simulink model "Master_compact"  (R2016b)
settings: Solver=FixedStepDiscrete  StartTime=0.0  StopTime=3000e-6  FixedStep=10e-9  RelTol=1e-3
undefined symbols (not defined in the file): plecs
libraries: hdlsllib x2, simulink x2, modelsimlib x1
settings Model: Creator=pzaehner  LastModifiedBy=pzaehner

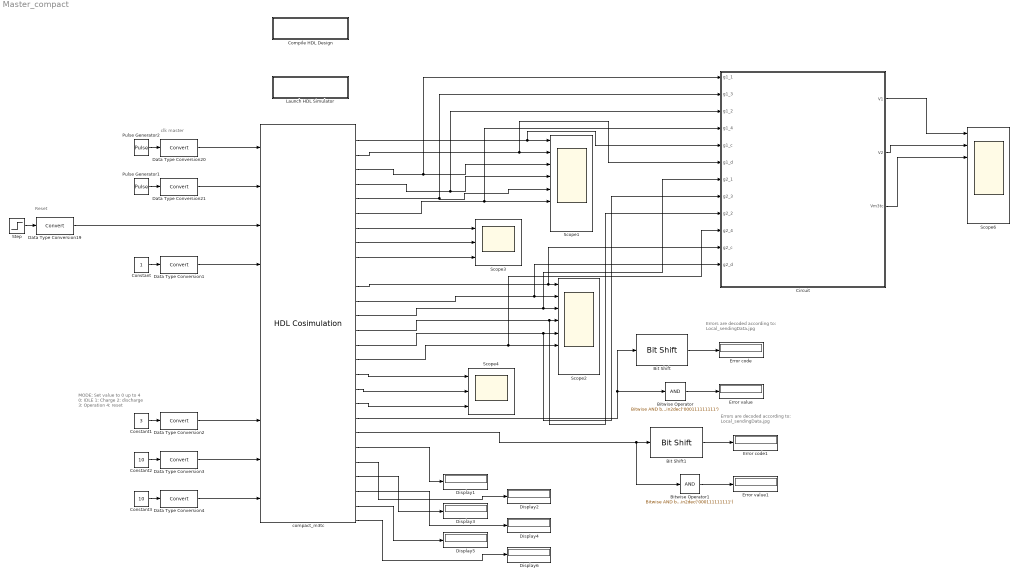
== system Master_compact ==
  note: clk master
  note: Reset
  note: MODE:
      | Set value to 0 up to 4
      | 0: IDLE
      | 1: Charge
      | 2: discharge
      | 3: Operation
      | 4: reset
  note: Errors are decoded according to:
      | Local_sendingData.jpg
  note: Errors are decoded according to:
      | Local_sendingData.jpg
  Bit Shift : hdlsllib/HDL Operations/Bit Shift  mode=Shift Right Logical  N=9
  Bit Shift1 : hdlsllib/HDL Operations/Bit Shift  mode=Shift Right Logical  N=9
  Bitwise Operator : simulink/Logic and Bit Operations/Bitwise Operator  logicop=AND  UseBitMask=on  BitMask=bin2dec('000111111111')  BitMaskRealWorld=Stored Integer
  Bitwise Operator1 : simulink/Logic and Bit Operations/Bitwise Operator  logicop=AND  UseBitMask=on  BitMask=bin2dec('000111111111')  BitMaskRealWorld=Stored Integer
  Circuit : Subsystem  LoadFcn=plecs('sl', 200);  InitFcn=plecs('sl', 214);  StartFcn=plecs('sl', 208);  StopFcn=plecs('sl', 209);  mask(PlecsCircuit){PLECSData=<binary blob, 7016 chars, not shown>}
      mask prompts: PLECSData "PLECS Data (Do not delete or modify!)"
      mask init:
      | % PLACE CUSTOM INITIALIZATIONS ABOVE
      | % DO NOT REMOVE
      | plecs('sl', 215);
      | % DO NOT REMOVE
      settings: CopyFcn=plecs('sl', 203);  DeleteFcn=plecs('sl', 205);  UndoDeleteFcn=plecs('sl', 206);  PreSaveFcn=plecs('sl', 211);  PostSaveFcn=plecs('sl', 201);  NameChangeFcn=plecs('sl', 210);  DestroyFcn=plecs('sl', 207);  PreCopyFcn=plecs('sl', 216);  OpenFcn=plecs('sl', 202);  ErrorFcn=plerrorfcn
      mask Help: web(['file:///' fullfile(plecsdoc, 'creatingacircuit.html')])
      mask Display: disp('PLECS\nCircuit')
  Compile HDL Design : Subsystem
      settings: OpenFcn=eval('compile_hdl_design_compact_m3tc');
      mask Display: disp(['Double-Click to' char(10) 'compile HDL files'])
  Constant : Constant  SampleTime=10e-9
  Constant1 : Constant  Value=3  SampleTime=10e-9
  Constant2 : Constant  Value=10  SampleTime=10e-9
  Constant3 : Constant  Value=10  SampleTime=10e-9
  Data Type Conversion{1..4,19..21} (7 alike) : DataTypeConversion
  Display{1..6} (6 alike) : Display
  Error code : Display
  Error code1 : Display
  Error value : Display
  Error value1 : Display
  Launch HDL Simulator : Subsystem
      settings: OpenFcn=eval('launch_hdl_simulator_compact_m3tc');
      mask Display: disp(['Double-Click to' char(10) 'launch HDL simulator'])
  Pulse Generator1 : DiscretePulseGenerator  PulseType=Time based  Period=20e-9  PulseWidth=50  PhaseDelay=10e-9
  Pulse Generator2 : DiscretePulseGenerator  PulseType=Time based  Period=20e-9  PulseWidth=50  PhaseDelay=10e-9
  Scope1 : Scope  NumInputPorts=8
  Scope2 : Scope  NumInputPorts=8
  Scope3 : Scope  NumInputPorts=3
  Scope4 : Scope  NumInputPorts=3
  Scope6 : Scope  NumInputPorts=8
  Step : Step  Time=100e-9  SampleTime=10e-9
  compact_m3tc : modelsimlib/HDL Cosimulation  PortPaths=/compact_m3tc/CLK_Master;/compact_m3tc/optical_Clk_1;/compact_m3tc/nreset;/compact_m3tc/HIGH_Input;/compact_m3tc/masterCurrentMeas;/compact_m3tc/masterCurrentRef;/compact_m3tc/masterVOLT;/compact_m3tc/MODE_put_to_3;/compact_m3tc/Number_12_bit3;/compact_m3tc/Number_8_bit;/compact_m3tc/optical_fault_1;/compact_m3tc/gate_c_1;/compact_m3tc/gate_d_1;/compact_m3tc/gate_1_1;/compact_m3tc/gate_2_1;/compact_m3tc/gate_3_1;/compact_m3tc/gate_4_1;/compact_m3tc/rst_c_1;/compact_m3tc/rst_d_1;/compact_m3tc/rst_overall_1;/compact_m3tc/optical_fault_2;/compact_m3tc/gate_c_2;/compact_m3tc/gate_d_2;/compact_m3tc/gate_1_2;/compact_m3tc/gate_2_2;/compact_m3tc/gate_3_2;/compact_m3tc/gate_4_2;/compact_m3tc/rst_c_2;/compact_m3tc/rst_d_2;/compact_m3tc/rst_overall_2;/compact_m3tc/outFAULT_1;/compact_m3tc/outFAULT_2;/compact_m3tc/outTempHS_1;/compact_m3tc/outTempHS_2;/compact_m3tc/outTempIGBT_1;/compact_m3tc/outTempIGBT_2;/compact_m3tc/outVOLT_1;/compact_m3tc/outVOLT_2;  PortModes=[1 1 1 1 1 1 1 1 1 1 2 2 2 2 2 2 2 2 2 2 2 2 2 2 2 2 2 2 2 2 2 2 2 2 2 2 2 2 ]  PortTimes=[-1,-1,-1,-1,-1,-1,-1,-1,-1,-1,10e-9,10e-9,10e-9,10e-9,10e-9,10e-9,10e-9,10e-9,10e-9,10e-9,10e-9,10e-9,10e-9,10e-9,10e-9,10e-9,10e-9,10e-9,10e-9,10e-9,10e-9,10e-9,10e-9,10e-9,10e-9,10e-9,10e-9,10e-9]  PortSigns=[-1,-1,-1,-1,-1,-1,-1,-1,-1,-1,-1,-1,-1,-1,-1,-1,-1,-1,-1,-1,-1,-1,-1,-1,-1,-1,-1,-1,-1,-1,-1,-1,-1,-1,-1,-1,-1,-1,]  PortFracLengths=[0,0,0,0,0,0,0,0,0,0,0,0,0,0,0,0,0,0,0,0,0,0,0,0,0,0,0,0,0,0,0,0,0,0,0,0,0,0]  CommLocal=on  CommSharedMemory=off  CommPortNumber=49294  CommShowInfo=on  ClockModes=[]  ClockTimes=[]  TclPostSimCommand="puts \"done\";"  TimingMode=s  TimingScaleFactor=1  idxCellArray={'UNUSED_VAR'}  CosimBypass=Full Simulation  AllowDirectFeedthrough=on  ProductName=EDA Simulator Link MQ  RunAutoTimescale=on  PreRunTime=0  PreRunTimeUnit=ns
  wires:
  Data Type Conversion19/1 -> compact_m3tc/3
  Step/1 -> Data Type Conversion19/1
  Pulse Generator2/1 -> Data Type Conversion20/1
  Pulse Generator1/1 -> Data Type Conversion21/1
  Data Type Conversion21/1 -> compact_m3tc/2
  Circuit/1(V1) -> Scope6/1
  Circuit/2(V2) -> Scope6/2
  Bit Shift/1 -> Error code/1
  Bitwise Operator/1 -> Error value/1
  Bit Shift1/1 -> Error code1/1
  Bitwise Operator1/1 -> Error value1/1
  compact_m3tc/22 -> Bitwise Operator1/1, Bit Shift1/1
  compact_m3tc/24 -> Display2/1
  compact_m3tc/27 -> Display5/1
  compact_m3tc/28 -> Display6/1
  compact_m3tc/26 -> Display4/1
  compact_m3tc/2 -> Circuit/5(g1_c), Scope1/1
  compact_m3tc/4 -> Circuit/1(g1_1), Scope1/3
  compact_m3tc/5 -> Circuit/3(g1_2), Scope1/4
  compact_m3tc/6 -> Scope1/5, Circuit/2(g1_3)
  compact_m3tc/7 -> Circuit/4(g1_4), Scope1/6
  compact_m3tc/12 -> Circuit/11(g2_c), Scope2/1
  compact_m3tc/14 -> Circuit/7(g2_1), Scope2/3
  compact_m3tc/15 -> Circuit/9(g2_2), Scope2/4
  compact_m3tc/16 -> Circuit/8(g2_3), Scope2/5
  compact_m3tc/17 -> Circuit/10(g2_4), Scope2/6
  compact_m3tc/18 -> Scope4/1
  compact_m3tc/19 -> Scope4/2
  compact_m3tc/20 -> Scope4/3
  compact_m3tc/21 -> Bitwise Operator/1, Bit Shift/1
  compact_m3tc/3 -> Circuit/6(g1_d), Scope1/2
  Circuit/3(Vm3tc) -> Scope6/3
  compact_m3tc/8 -> Scope3/1
  compact_m3tc/9 -> Scope3/2
  compact_m3tc/10 -> Scope3/3
  compact_m3tc/13 -> Circuit/12(g2_d), Scope2/2
  compact_m3tc/23 -> Display1/1
  compact_m3tc/25 -> Display3/1
  Data Type Conversion20/1 -> compact_m3tc/1
  Data Type Conversion1/1 -> compact_m3tc/4
  Constant/1 -> Data Type Conversion1/1
  Data Type Conversion2/1 -> compact_m3tc/8
  Constant1/1 -> Data Type Conversion2/1
  Data Type Conversion3/1 -> compact_m3tc/9
  Constant2/1 -> Data Type Conversion3/1
  Data Type Conversion4/1 -> compact_m3tc/10
  Constant3/1 -> Data Type Conversion4/1

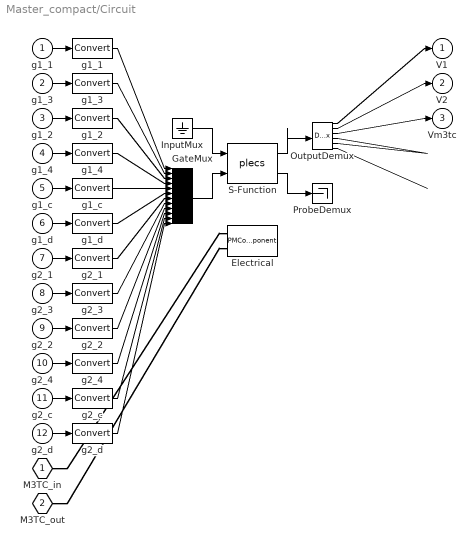
== system Master_compact/Circuit ==
  g1_1 : Inport  PortDimensions=1
  g1_3 : Inport  Port=2  PortDimensions=1
  g1_2 : Inport  Port=3  PortDimensions=1
  g1_4 : Inport  Port=4  PortDimensions=1
  g1_c : Inport  Port=5  PortDimensions=1
  g1_d : Inport  Port=6  PortDimensions=1
  g2_1 : Inport  Port=7  PortDimensions=1
  g2_3 : Inport  Port=8  PortDimensions=1
  g2_2 : Inport  Port=9  PortDimensions=1
  g2_4 : Inport  Port=10  PortDimensions=1
  g2_c : Inport  Port=11  PortDimensions=1
  g2_d : Inport  Port=12  PortDimensions=1
  " Electrical " : PMComponent  PhysicalDomain=plecsdomain  LeftPortType=electrical  RightPortType=blob  LConnTagsString=__newl1|__newl2
  " GateMux " : Mux  Inputs=[ 1 1 1 1 1 1 1 1 1 1 1 1 ]
  " InputMux " : Ground
  " OutputDemux " : Demux  Outputs=[ 1 1 1 1 1 1 ]
  " ProbeDemux " : Terminator
  " S-Function " : S-Function  FunctionName=plecs  SFunctionDeploymentMode=off  EnableBusSupport=off
  " g1_1 " : DataTypeConversion  SaturateOnIntegerOverflow=on  RndMeth=Zero
  " g1_2 " : DataTypeConversion  SaturateOnIntegerOverflow=on  RndMeth=Zero
  " g1_3 " : DataTypeConversion  SaturateOnIntegerOverflow=on  RndMeth=Zero
  " g1_4 " : DataTypeConversion  SaturateOnIntegerOverflow=on  RndMeth=Zero
  " g1_c " : DataTypeConversion  SaturateOnIntegerOverflow=on  RndMeth=Zero
  " g1_d " : DataTypeConversion  SaturateOnIntegerOverflow=on  RndMeth=Zero
  " g2_1 " : DataTypeConversion  SaturateOnIntegerOverflow=on  RndMeth=Zero
  " g2_2 " : DataTypeConversion  SaturateOnIntegerOverflow=on  RndMeth=Zero
  " g2_3 " : DataTypeConversion  SaturateOnIntegerOverflow=on  RndMeth=Zero
  " g2_4 " : DataTypeConversion  SaturateOnIntegerOverflow=on  RndMeth=Zero
  " g2_c " : DataTypeConversion  SaturateOnIntegerOverflow=on  RndMeth=Zero
  " g2_d " : DataTypeConversion  SaturateOnIntegerOverflow=on  RndMeth=Zero
  M3TC_in : PMIOPort  Port=1  Side=Left
  M3TC_out : PMIOPort  Port=2  Side=Right
  V1 : Outport  PortDimensions=1
  V2 : Outport  Port=2  PortDimensions=1
  Vm3tc : Outport  Port=3  PortDimensions=1
  wires:
  " S-Function "/1 -> " OutputDemux "/1
  " InputMux "/1 -> " S-Function "/1
  " GateMux "/1 -> " S-Function "/2
  " S-Function "/2 -> " ProbeDemux "/1
  g1_1/1 -> " g1_1 "/1
  " g1_1 "/1 -> " GateMux "/1
  g1_3/1 -> " g1_3 "/1
  " g1_3 "/1 -> " GateMux "/2
  g1_2/1 -> " g1_2 "/1
  " g1_2 "/1 -> " GateMux "/3
  g1_4/1 -> " g1_4 "/1
  " g1_4 "/1 -> " GateMux "/4
  g1_c/1 -> " g1_c "/1
  " g1_c "/1 -> " GateMux "/5
  g1_d/1 -> " g1_d "/1
  " g1_d "/1 -> " GateMux "/6
  g2_1/1 -> " g2_1 "/1
  " g2_1 "/1 -> " GateMux "/7
  g2_3/1 -> " g2_3 "/1
  " g2_3 "/1 -> " GateMux "/8
  g2_2/1 -> " g2_2 "/1
  " g2_2 "/1 -> " GateMux "/9
  g2_4/1 -> " g2_4 "/1
  " g2_4 "/1 -> " GateMux "/10
  g2_c/1 -> " g2_c "/1
  " g2_c "/1 -> " GateMux "/11
  g2_d/1 -> " g2_d "/1
  " g2_d "/1 -> " GateMux "/12
  " OutputDemux "/1 -> V1/1
  " OutputDemux "/2 -> V2/1
  " OutputDemux "/3 -> Vm3tc/1
  " OutputDemux "/4 -> ?
  " OutputDemux "/5 -> ?
  " OutputDemux "/6 -> ?
  connections:
  M3TC_in/RConn1 -- " Electrical "/LConn1
  M3TC_out/RConn1 -- " Electrical "/LConn2

== system Master_compact/Compile HDL Design ==

== system Master_compact/Launch HDL Simulator ==
